simulink model "HCSG_ss"  (R2018a)
settings: Solver=ode23t  StartTime=0.0  StopTime=1000  MaxStep=0.1  RelTol=1e-6
values from neighbouring files (symbols this model uses):
  a_11 = A_s*Cp_sc*rho_sc/2    (= 0.000255426988715)    [MSDR_parameters.m]
  a_12 = h_wsc*pi*R_i/a_2    (= 0.891425789979)    [MSDR_parameters.m]
  a_13 = h_wsc*pi*R_i/a_11    (= 0.682722842114)    [MSDR_parameters.m]
  a_3 = A_s*Cp_s*rho_s/2    [MSDR_parameters.m]
  a_4 = h_pw*pi*R_o/a_1    (= 0.0704483418498)    [MSDR_parameters.m]
  a_51 = Cp_p*W_p0/a_1    (= 1.13472152802)    [MSDR_parameters.m]
  a_52 = Cp_p*W_p1/a_1    (= 1.13472152802)    [MSDR_parameters.m]
  a_53 = Cp_p*W_p2/a_1    (= 1.13472152802)    [MSDR_parameters.m]
  a_54 = Cp_p*W_p3/a_1    (= 1.13472152802)    [MSDR_parameters.m]
  a_55 = Cp_p*W_p4/a_1    (= 1.13472152802)    [MSDR_parameters.m]
  a_56 = Cp_p*W_p5/a_1    (= 1.13472152802)    [MSDR_parameters.m]
  a_6 = h_pw*pi*R_o/a_2    (= 1.27597922538)    [MSDR_parameters.m]
  a_7 = h_wb*pi*R_i/a_2    (= 1.41919299911)    [MSDR_parameters.m]
  a_8 = h_ws*pi*R_i/a_2    (= 0.609419981706)    [MSDR_parameters.m]
  a_9 = h_ws*pi*R_i/a_3    [MSDR_parameters.m]
  Cp_fw = 4697.58960001e-6    (= 0.00469758960001)    [MSDR_parameters.m]
  Cp_s = Cp_s*1e-6    [MSDR_parameters.m]
  L_b = 21.5    [MSDR_parameters.m]
  L_s = L - L_b - L_sc    (= 6)    [MSDR_parameters.m]
  L_sc = 4.5    [MSDR_parameters.m]
  T_fw = 224    [MSDR_parameters.m]
  T_pin = 328.4    [MSDR_parameters.m]
  T_sat = X_5 + K_5*P_sat    [MSDR_parameters.m]
  W_b = W_sec    (= 0.0766463414634)    [MSDR_parameters.m]
  W_fw = W_sec    (= 0.0766463414634)    [MSDR_parameters.m]
  W_s = W_sec    (= 0.0766463414634)    [MSDR_parameters.m]
settings Model: Creator=viikr  LastModifiedBy=viikr

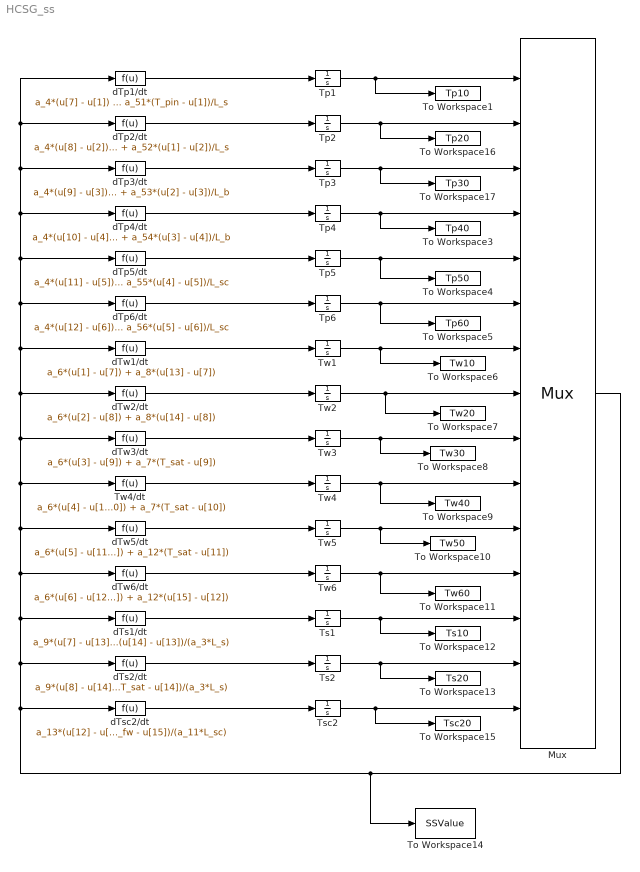
== system HCSG_ss ==
  Mux : Mux  Inputs=15
      settings: DisplayOption=signals
  To Workspace1 : ToWorkspace  VariableName=Tp10  SampleTime=-1
  To Workspace10 : ToWorkspace  VariableName=Tw50  SampleTime=-1
  To Workspace11 : ToWorkspace  VariableName=Tw60  SampleTime=-1
  To Workspace12 : ToWorkspace  VariableName=Ts10  SampleTime=-1
  To Workspace13 : ToWorkspace  VariableName=Ts20  SampleTime=-1
  To Workspace14 : ToWorkspace  VariableName=SSValue  SampleTime=-1
  To Workspace15 : ToWorkspace  VariableName=Tsc20  SampleTime=-1
  To Workspace16 : ToWorkspace  VariableName=Tp20  SampleTime=-1
  To Workspace17 : ToWorkspace  VariableName=Tp30  SampleTime=-1
  To Workspace3 : ToWorkspace  VariableName=Tp40  SampleTime=-1
  To Workspace4 : ToWorkspace  VariableName=Tp50  SampleTime=-1
  To Workspace5 : ToWorkspace  VariableName=Tp60  SampleTime=-1
  To Workspace6 : ToWorkspace  VariableName=Tw10  SampleTime=-1
  To Workspace7 : ToWorkspace  VariableName=Tw20  SampleTime=-1
  To Workspace8 : ToWorkspace  VariableName=Tw30  SampleTime=-1
  To Workspace9 : ToWorkspace  VariableName=Tw40  SampleTime=-1
  Tp{1..6} (6 alike) : Integrator  InitialCondition=0.0
  Ts1 : Integrator  InitialCondition=0.0
  Ts2 : Integrator  InitialCondition=0.0
  Tsc2 : Integrator  InitialCondition=0.0
  Tw{1..6} (6 alike) : Integrator  InitialCondition=0.0
  Tw4/dt : Fcn  Expr=a_6*(u[4] - u[10]) + a_7*(T_sat - u[10])
  dTp1/dt : Fcn  Expr=a_4*(u[7] - u[1]) + a_51*(T_pin - u[1])/L_s
  dTp2/dt : Fcn  Expr=a_4*(u[8] - u[2]) + a_52*(u[1] - u[2])/L_s
  dTp3/dt : Fcn  Expr=a_4*(u[9] - u[3]) + a_53*(u[2] - u[3])/L_b
  dTp4/dt : Fcn  Expr=a_4*(u[10] - u[4]) + a_54*(u[3] - u[4])/L_b
  dTp5/dt : Fcn  Expr=a_4*(u[11] - u[5]) + a_55*(u[4] - u[5])/L_sc
  dTp6/dt : Fcn  Expr=a_4*(u[12] - u[6]) + a_56*(u[5] - u[6])/L_sc
  dTs1/dt : Fcn  Expr=a_9*(u[7] - u[13]) + W_s*Cp_s*(u[14] - u[13])/(a_3*L_s)
  dTs2/dt : Fcn  Expr=a_9*(u[8] - u[14]) + W_b*Cp_s*(T_sat - u[14])/(a_3*L_s)
  dTsc2/dt : Fcn  Expr=a_13*(u[12] - u[15]) + W_fw*Cp_fw*(T_fw - u[15])/(a_11*L_sc)
  dTw1/dt : Fcn  Expr=a_6*(u[1] - u[7]) + a_8*(u[13] - u[7])
  dTw2/dt : Fcn  Expr=a_6*(u[2] - u[8]) + a_8*(u[14] - u[8])
  dTw3/dt : Fcn  Expr=a_6*(u[3] - u[9]) + a_7*(T_sat - u[9])
  dTw5/dt : Fcn  Expr=a_6*(u[5] - u[11]) + a_12*(T_sat - u[11])
  dTw6/dt : Fcn  Expr=a_6*(u[6] - u[12]) + a_12*(u[15] - u[12])
  wires:
  Ts1/1 -> Mux/13, To Workspace12/1
  dTw5/dt/1 -> Tw5/1
  Tp3/1 -> Mux/3, To Workspace17/1
  Tsc2/1 -> Mux/15, To Workspace15/1
  Tw4/dt/1 -> Tw4/1
  dTsc2/dt/1 -> Tsc2/1
  Tw5/1 -> To Workspace10/1, Mux/11
  dTs2/dt/1 -> Ts2/1
  Tp4/1 -> Mux/4, To Workspace3/1
  dTp2/dt/1 -> Tp2/1
  Tw1/1 -> To Workspace6/1, Mux/7
  Tw6/1 -> To Workspace11/1, Mux/12
  dTp5/dt/1 -> Tp5/1
  Tw2/1 -> To Workspace7/1, Mux/8
  dTp4/dt/1 -> Tp4/1
  dTw1/dt/1 -> Tw1/1
  Tw3/1 -> To Workspace8/1, Mux/9
  Mux/1 -> dTsc2/dt/1, dTp1/dt/1, dTp2/dt/1, dTp3/dt/1, dTp4/dt/1, dTp5/dt/1, dTp6/dt/1, dTw1/dt/1, dTw2/dt/1, dTw3/dt/1, Tw4/dt/1, dTw5/dt/1, dTw6/dt/1, dTs1/dt/1, dTs2/dt/1, To Workspace14/1
  dTw6/dt/1 -> Tw6/1
  Tp2/1 -> Mux/2, To Workspace16/1
  dTw3/dt/1 -> Tw3/1
  Tp6/1 -> Mux/6, To Workspace5/1
  Tw4/1 -> To Workspace9/1, Mux/10
  dTp6/dt/1 -> Tp6/1
  dTp3/dt/1 -> Tp3/1
  Tp5/1 -> To Workspace4/1, Mux/5
  Tp1/1 -> Mux/1, To Workspace1/1
  Ts2/1 -> Mux/14, To Workspace13/1
  dTp1/dt/1 -> Tp1/1
  dTw2/dt/1 -> Tw2/1
  dTs1/dt/1 -> Ts1/1
